simulink model "ShubhamGupta_180749_LabExam_model"  (R2020b)
settings: Solver=VariableStepAuto  StartTime=0.0  StopTime=50  RelTol=1e-3
settings Model: Creator=subhamgupta  LastModifiedBy=subhamgupta
settings DataIOCC: ReturnWorkspaceOutputs=off

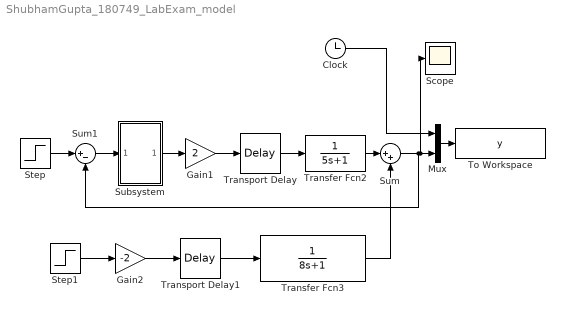
== system ShubhamGupta_180749_LabExam_model ==
  Clock : Clock
  Gain1 : Gain  Gain=2
  Gain2 : Gain  Gain=-2
  Mux : Mux  Inputs=2
  Scope : Scope
  Step : Step  Time=0  After=0  SampleTime=0
  Step1 : Step  SampleTime=0
  Subsystem : Subsystem  mask{kc=1.7527, ti=5, td=0}
      mask prompts: kc "Controller gain"; ti "integral time constant"; td "derivative time constant"
  Sum : Sum  Inputs=|++
  Sum1 : Sum  Inputs=|+-
  To Workspace : ToWorkspace  VariableName=y  SampleTime=-1
  Transfer Fcn2 : TransferFcn  Numerator=[0 1]  Denominator=[5 1]
  Transfer Fcn3 : TransferFcn  Numerator=[0 1]  Denominator=[8 1]
  Transport Delay : TransportDelay
  Transport Delay1 : TransportDelay  DelayTime=2
  wires:
  Gain1/1 -> Transport Delay/1
  Transport Delay/1 -> Transfer Fcn2/1
  Transfer Fcn2/1 -> Sum/1
  Sum/1 -> Sum1/2, Scope/1, Mux/2
  Transport Delay1/1 -> Transfer Fcn3/1
  Gain2/1 -> Transport Delay1/1
  Transfer Fcn3/1 -> Sum/2
  Step/1 -> Sum1/1
  Step1/1 -> Gain2/1
  Sum1/1 -> Subsystem/1(In1)
  Subsystem/1(Out1) -> Gain1/1
  Clock/1 -> Mux/1
  Mux/1 -> To Workspace/1

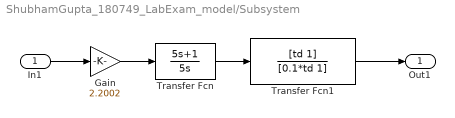
== system ShubhamGupta_180749_LabExam_model/Subsystem ==
  In1 : Inport
  Gain : Gain  Gain=2.2002
  Transfer Fcn : TransferFcn  Numerator=[5 1]  Denominator=[5 0]
  Transfer Fcn1 : TransferFcn  Numerator=[td 1]  Denominator=[0.1*td 1]
  Out1 : Outport
  wires:
  In1/1 -> Gain/1
  Transfer Fcn1/1 -> Out1/1
  Transfer Fcn/1 -> Transfer Fcn1/1
  Gain/1 -> Transfer Fcn/1
